simulink model "Exp1_Unipolar_Polar_RZ"  (R2020b)
settings: Solver=VariableStepAuto  StartTime=0.0  StopTime=10.0  RelTol=1e-3
libraries: commrandsrc3 x1
settings Model: Creator=Mohit Akhouri  LastModifiedBy=Mohit Akhouri

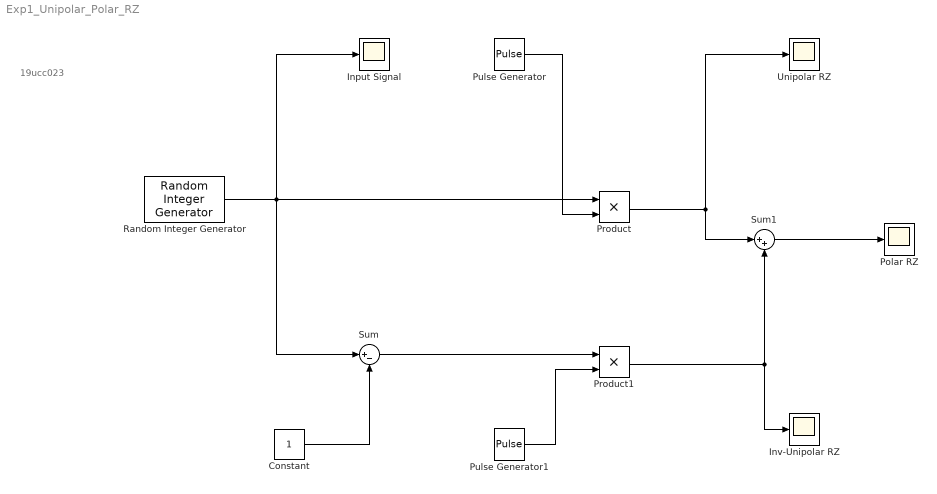
== system Exp1_Unipolar_Polar_RZ ==
  note: 19ucc023
  Constant : Constant
  Input Signal : Scope
  Inv-Unipolar RZ : Scope
  Polar RZ : Scope
  Product : Product
  Product1 : Product
  Pulse Generator : DiscretePulseGenerator  PulseType=Time based  Period=1  PulseWidth=50
  Pulse Generator1 : DiscretePulseGenerator  PulseType=Time based  Period=1  PulseWidth=50
  Random Integer Generator : commrandsrc3/Random Integer Generator  SetSize=2  SeedSource=Parameter  Seed=0  SampleTime=1  SamplesPerFrame=1  OutputDataType=double  SimulateUsing=Interpreted execution
  Sum : Sum  Inputs=|+-
  Sum1 : Sum  Inputs=|++
  Unipolar RZ : Scope
  wires:
  Random Integer Generator/1 -> Input Signal/1, Product/1, Sum/1
  Pulse Generator/1 -> Product/2
  Constant/1 -> Sum/2
  Sum/1 -> Product1/1
  Pulse Generator1/1 -> Product1/2
  Product/1 -> Sum1/1, Unipolar RZ/1
  Product1/1 -> Inv-Unipolar RZ/1, Sum1/2
  Sum1/1 -> Polar RZ/1
